simulink library "inSOMANET"  (R2016b)
settings: Solver=VariableStepAuto  StartTime=0.0  StopTime=10.0  RelTol=1e-3
libraries: ConversionsLibrary x28, xpcethercatlib x12
settings Model: Creator=Nathan  LastModifiedBy=MARCH

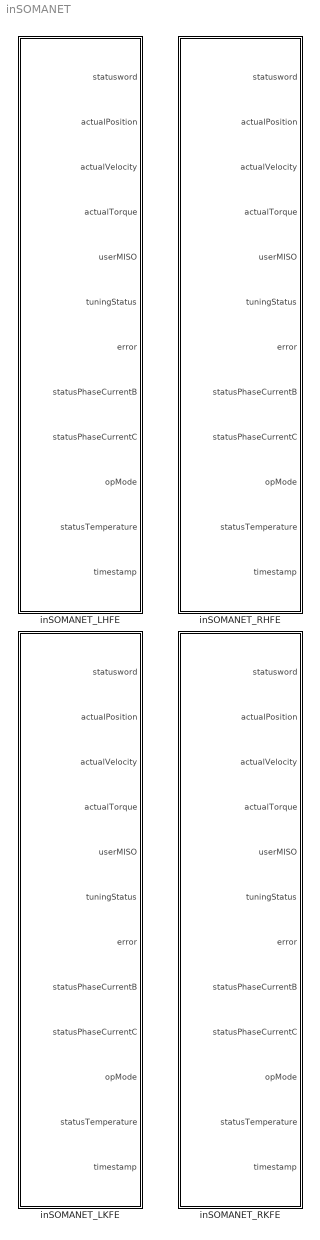
== system inSOMANET ==
  inSOMANET_LHFE : Subsystem
  inSOMANET_LKFE : Subsystem
  inSOMANET_RHFE : Subsystem
  inSOMANET_RKFE : Subsystem

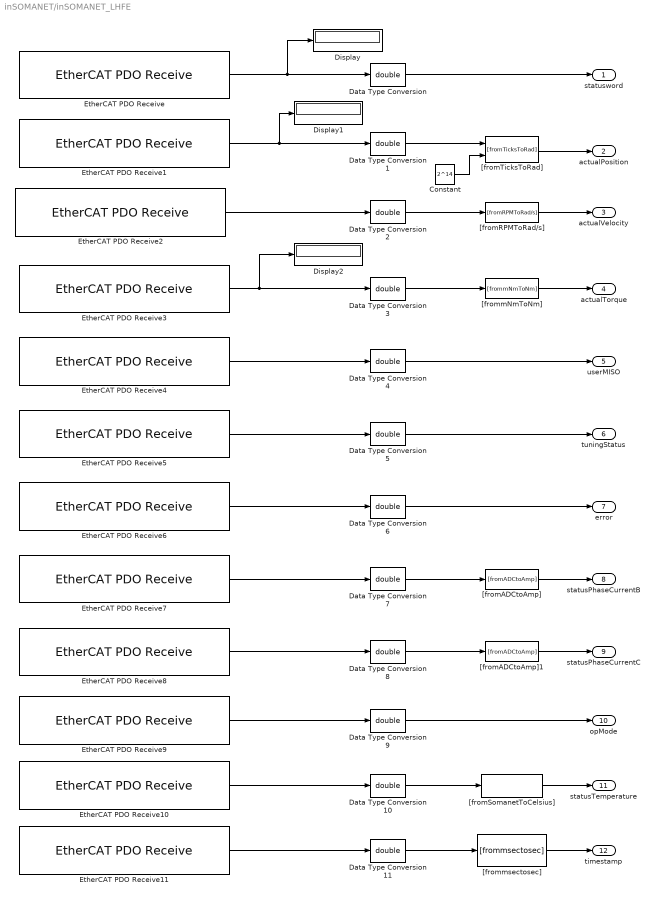
== system inSOMANET/inSOMANET_LHFE ==
  Constant : Constant  Value=2^14
  Data Type Conversion{,1..11} (12 alike) : DataTypeConversion  OutDataTypeStr=double
  Display : Display
  Display1 : Display
  Display2 : Display
  EtherCAT PDO Receive : xpcethercatlib/EtherCAT PDO Receive  Priority=2  sig_name=Drive 1 (CiA402 Motor Control Device).Inputs.Statusword  sig_offset=208  sig_type=uint16  type_size=16  sig_dim=1  device_id=0  sample_time=0.002000
  EtherCAT PDO Receive1 : xpcethercatlib/EtherCAT PDO Receive  Priority=2  sig_name=Drive 1 (CiA402 Motor Control Device).Inputs.Position Value  sig_offset=232  sig_type=int32  type_size=32  sig_dim=1  device_id=0  sample_time=0.002000
  EtherCAT PDO Receive10 : xpcethercatlib/EtherCAT PDO Receive  Priority=2  sig_name=Drive 1 (CiA402 Motor Control Device).Inputs.Core temperature  sig_offset=616  sig_type=int16  type_size=16  sig_dim=1  device_id=0  sample_time=0.002000
  EtherCAT PDO Receive11 : xpcethercatlib/EtherCAT PDO Receive  Priority=2  sig_name=Drive 1 (CiA402 Motor Control Device).Inputs.Timestamp  sig_offset=536  sig_type=uint32  type_size=32  sig_dim=1  device_id=0  sample_time=0.002000
  EtherCAT PDO Receive2 : xpcethercatlib/EtherCAT PDO Receive  Priority=2  sig_name=Drive 1 (CiA402 Motor Control Device).Inputs.Velocity Value  sig_offset=264  sig_type=int32  type_size=32  sig_dim=1  device_id=0  sample_time=0.002000
  EtherCAT PDO Receive3 : xpcethercatlib/EtherCAT PDO Receive  Priority=2  sig_name=Drive 1 (CiA402 Motor Control Device).Inputs.Torque Value  sig_offset=296  sig_type=int16  type_size=16  sig_dim=1  device_id=0  sample_time=0.002000
  EtherCAT PDO Receive4 : xpcethercatlib/EtherCAT PDO Receive  Priority=2  sig_name=Drive 1 (CiA402 Motor Control Device).Inputs.User MISO  sig_offset=504  sig_type=uint32  type_size=32  sig_dim=1  device_id=0  sample_time=0.002000
  EtherCAT PDO Receive5 : xpcethercatlib/EtherCAT PDO Receive  Priority=2  sig_name=Drive 1 (CiA402 Motor Control Device).Inputs.Tuning status  sig_offset=440  sig_type=uint32  type_size=32  sig_dim=1  device_id=0  sample_time=0.002000
  EtherCAT PDO Receive6 : xpcethercatlib/EtherCAT PDO Receive  Priority=2  sig_name=Drive 1 (CiA402 Motor Control Device).Inputs.Error code  sig_offset=568  sig_type=uint16  type_size=16  sig_dim=1  device_id=0  sample_time=0.002000
  EtherCAT PDO Receive7 : xpcethercatlib/EtherCAT PDO Receive  Priority=2  sig_name=Drive 1 (CiA402 Motor Control Device).Inputs.Instantaneous Phase B current  sig_offset=584  sig_type=int16  type_size=16  sig_dim=1  device_id=0  sample_time=0.002000
  EtherCAT PDO Receive8 : xpcethercatlib/EtherCAT PDO Receive  Priority=2  sig_name=Drive 1 (CiA402 Motor Control Device).Inputs.Instantaneous Phase C current  sig_offset=600  sig_type=int16  type_size=16  sig_dim=1  device_id=0  sample_time=0.002000
  EtherCAT PDO Receive9 : xpcethercatlib/EtherCAT PDO Receive  Priority=2  sig_name=Drive 1 (CiA402 Motor Control Device).Inputs.Op Mode Display  sig_offset=224  sig_type=int8  type_size=8  sig_dim=1  device_id=0  sample_time=0.002000
  "[fromADCtoAmp]" : ConversionsLibrary/[fromADCtoAmp]
  "[fromADCtoAmp]1" : ConversionsLibrary/[fromADCtoAmp]
  "[fromRPMToRad/s]" : ConversionsLibrary/[fromRPMToRad//s]
  "[fromSomanetToCelsius]" : ConversionsLibrary/[fromSomanetToCelsius]
  "[fromTicksToRad]" : ConversionsLibrary/[fromTicksToRad]
  "[frommNmToNm]" : ConversionsLibrary/[frommNmToNm]
  "[frommsectosec]" : ConversionsLibrary/[frommsectosec]
  statusword : Outport
  actualPosition : Outport  Port=2
  actualVelocity : Outport  Port=3
  actualTorque : Outport  Port=4
  userMISO : Outport  Port=5
  tuningStatus : Outport  Port=6
  error : Outport  Port=7
  statusPhaseCurrentB : Outport  Port=8
  statusPhaseCurrentC : Outport  Port=9
  opMode : Outport  Port=10
  statusTemperature : Outport  Port=11
  timestamp : Outport  Port=12
  wires:
  EtherCAT PDO Receive11/1 -> Data Type Conversion11/1
  EtherCAT PDO Receive10/1 -> Data Type Conversion10/1
  EtherCAT PDO Receive9/1 -> Data Type Conversion9/1
  EtherCAT PDO Receive8/1 -> Data Type Conversion8/1
  EtherCAT PDO Receive7/1 -> Data Type Conversion7/1
  EtherCAT PDO Receive6/1 -> Data Type Conversion6/1
  EtherCAT PDO Receive5/1 -> Data Type Conversion5/1
  EtherCAT PDO Receive4/1 -> Data Type Conversion4/1
  EtherCAT PDO Receive3/1 -> Data Type Conversion3/1, Display2/1
  EtherCAT PDO Receive2/1 -> Data Type Conversion2/1
  EtherCAT PDO Receive1/1 -> Data Type Conversion1/1, Display1/1
  EtherCAT PDO Receive/1 -> Data Type Conversion/1, Display/1
  Data Type Conversion/1 -> statusword/1
  Data Type Conversion11/1 -> "[frommsectosec]"/1
  Data Type Conversion10/1 -> "[fromSomanetToCelsius]"/1
  Data Type Conversion9/1 -> opMode/1
  Data Type Conversion8/1 -> "[fromADCtoAmp]1"/1
  Data Type Conversion7/1 -> "[fromADCtoAmp]"/1
  Data Type Conversion6/1 -> error/1
  Data Type Conversion5/1 -> tuningStatus/1
  Data Type Conversion4/1 -> userMISO/1
  Data Type Conversion3/1 -> "[frommNmToNm]"/1
  Data Type Conversion2/1 -> "[fromRPMToRad/s]"/1
  "[frommsectosec]"/1 -> timestamp/1
  "[fromSomanetToCelsius]"/1 -> statusTemperature/1
  "[fromADCtoAmp]1"/1 -> statusPhaseCurrentC/1
  "[fromADCtoAmp]"/1 -> statusPhaseCurrentB/1
  "[frommNmToNm]"/1 -> actualTorque/1
  "[fromRPMToRad/s]"/1 -> actualVelocity/1
  "[fromTicksToRad]"/1 -> actualPosition/1
  Data Type Conversion1/1 -> "[fromTicksToRad]"/1
  Constant/1 -> "[fromTicksToRad]"/2

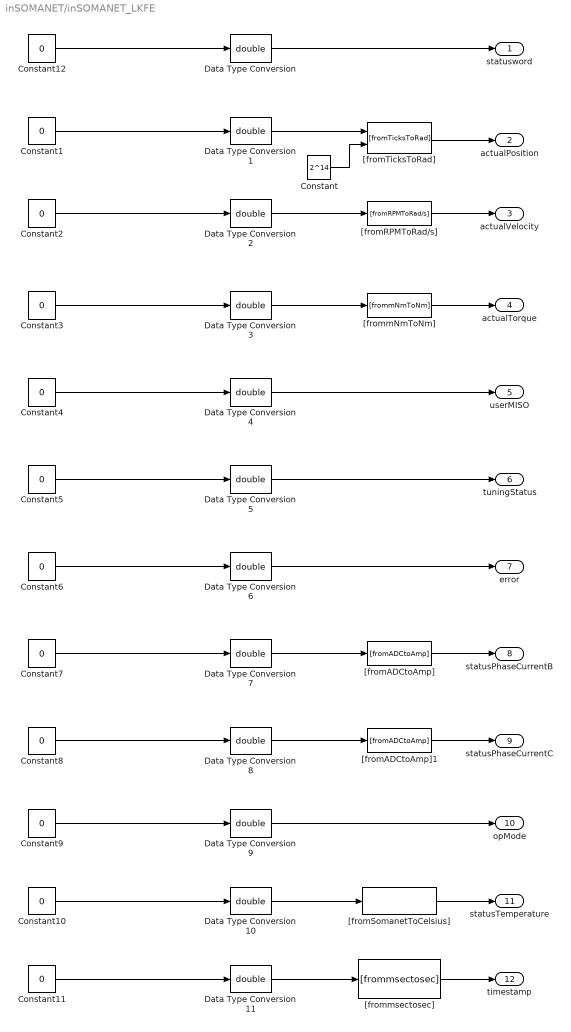
== system inSOMANET/inSOMANET_LKFE ==
  Constant : Constant  Value=2^14
  Constant{1..12} (12 alike) : Constant  Value=0
  Data Type Conversion{,1..11} (12 alike) : DataTypeConversion  OutDataTypeStr=double
  "[fromADCtoAmp]" : ConversionsLibrary/[fromADCtoAmp]
  "[fromADCtoAmp]1" : ConversionsLibrary/[fromADCtoAmp]
  "[fromRPMToRad/s]" : ConversionsLibrary/[fromRPMToRad//s]
  "[fromSomanetToCelsius]" : ConversionsLibrary/[fromSomanetToCelsius]
  "[fromTicksToRad]" : ConversionsLibrary/[fromTicksToRad]
  "[frommNmToNm]" : ConversionsLibrary/[frommNmToNm]
  "[frommsectosec]" : ConversionsLibrary/[frommsectosec]
  statusword : Outport
  actualPosition : Outport  Port=2
  actualVelocity : Outport  Port=3
  actualTorque : Outport  Port=4
  userMISO : Outport  Port=5
  tuningStatus : Outport  Port=6
  error : Outport  Port=7
  statusPhaseCurrentB : Outport  Port=8
  statusPhaseCurrentC : Outport  Port=9
  opMode : Outport  Port=10
  statusTemperature : Outport  Port=11
  timestamp : Outport  Port=12
  wires:
  Constant11/1 -> Data Type Conversion11/1
  Constant10/1 -> Data Type Conversion10/1
  Constant9/1 -> Data Type Conversion9/1
  Constant8/1 -> Data Type Conversion8/1
  Constant7/1 -> Data Type Conversion7/1
  Constant6/1 -> Data Type Conversion6/1
  Constant5/1 -> Data Type Conversion5/1
  Constant4/1 -> Data Type Conversion4/1
  Constant3/1 -> Data Type Conversion3/1
  Constant2/1 -> Data Type Conversion2/1
  Constant1/1 -> Data Type Conversion1/1
  Constant12/1 -> Data Type Conversion/1
  Data Type Conversion/1 -> statusword/1
  Data Type Conversion11/1 -> "[frommsectosec]"/1
  Data Type Conversion10/1 -> "[fromSomanetToCelsius]"/1
  Data Type Conversion9/1 -> opMode/1
  Data Type Conversion8/1 -> "[fromADCtoAmp]1"/1
  Data Type Conversion7/1 -> "[fromADCtoAmp]"/1
  Data Type Conversion6/1 -> error/1
  Data Type Conversion5/1 -> tuningStatus/1
  Data Type Conversion4/1 -> userMISO/1
  Data Type Conversion3/1 -> "[frommNmToNm]"/1
  Data Type Conversion2/1 -> "[fromRPMToRad/s]"/1
  "[frommsectosec]"/1 -> timestamp/1
  "[fromSomanetToCelsius]"/1 -> statusTemperature/1
  "[fromADCtoAmp]1"/1 -> statusPhaseCurrentC/1
  "[fromADCtoAmp]"/1 -> statusPhaseCurrentB/1
  "[frommNmToNm]"/1 -> actualTorque/1
  "[fromRPMToRad/s]"/1 -> actualVelocity/1
  "[fromTicksToRad]"/1 -> actualPosition/1
  Data Type Conversion1/1 -> "[fromTicksToRad]"/1
  Constant/1 -> "[fromTicksToRad]"/2

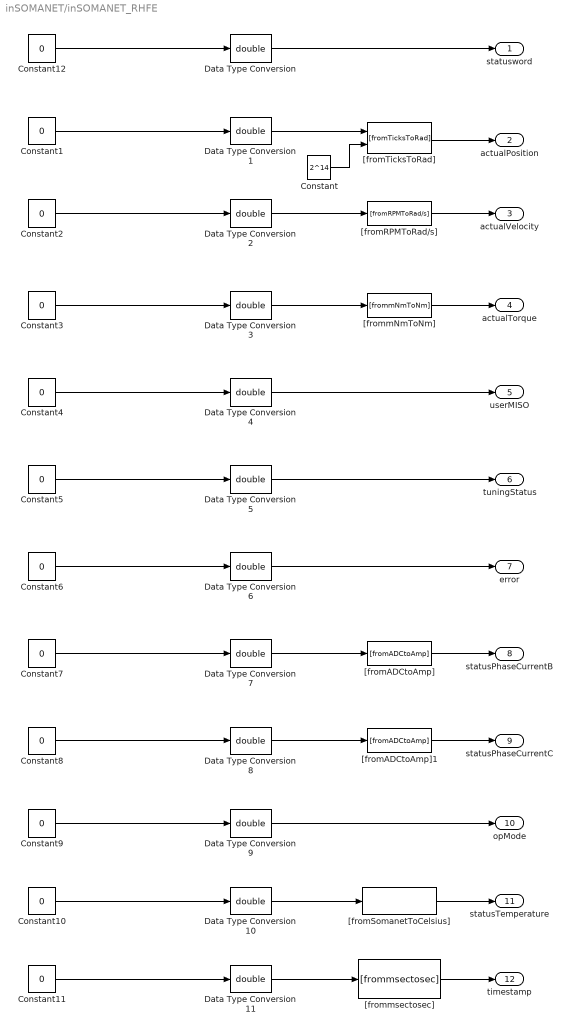
== system inSOMANET/inSOMANET_RHFE ==
  Constant : Constant  Value=2^14
  Constant{1..12} (12 alike) : Constant  Value=0
  Data Type Conversion{,1..11} (12 alike) : DataTypeConversion  OutDataTypeStr=double
  "[fromADCtoAmp]" : ConversionsLibrary/[fromADCtoAmp]
  "[fromADCtoAmp]1" : ConversionsLibrary/[fromADCtoAmp]
  "[fromRPMToRad/s]" : ConversionsLibrary/[fromRPMToRad//s]
  "[fromSomanetToCelsius]" : ConversionsLibrary/[fromSomanetToCelsius]
  "[fromTicksToRad]" : ConversionsLibrary/[fromTicksToRad]
  "[frommNmToNm]" : ConversionsLibrary/[frommNmToNm]
  "[frommsectosec]" : ConversionsLibrary/[frommsectosec]
  statusword : Outport
  actualPosition : Outport  Port=2
  actualVelocity : Outport  Port=3
  actualTorque : Outport  Port=4
  userMISO : Outport  Port=5
  tuningStatus : Outport  Port=6
  error : Outport  Port=7
  statusPhaseCurrentB : Outport  Port=8
  statusPhaseCurrentC : Outport  Port=9
  opMode : Outport  Port=10
  statusTemperature : Outport  Port=11
  timestamp : Outport  Port=12
  wires:
  Constant11/1 -> Data Type Conversion11/1
  Constant10/1 -> Data Type Conversion10/1
  Constant9/1 -> Data Type Conversion9/1
  Constant8/1 -> Data Type Conversion8/1
  Constant7/1 -> Data Type Conversion7/1
  Constant6/1 -> Data Type Conversion6/1
  Constant5/1 -> Data Type Conversion5/1
  Constant4/1 -> Data Type Conversion4/1
  Constant3/1 -> Data Type Conversion3/1
  Constant2/1 -> Data Type Conversion2/1
  Constant1/1 -> Data Type Conversion1/1
  Constant12/1 -> Data Type Conversion/1
  Data Type Conversion/1 -> statusword/1
  Data Type Conversion11/1 -> "[frommsectosec]"/1
  Data Type Conversion10/1 -> "[fromSomanetToCelsius]"/1
  Data Type Conversion9/1 -> opMode/1
  Data Type Conversion8/1 -> "[fromADCtoAmp]1"/1
  Data Type Conversion7/1 -> "[fromADCtoAmp]"/1
  Data Type Conversion6/1 -> error/1
  Data Type Conversion5/1 -> tuningStatus/1
  Data Type Conversion4/1 -> userMISO/1
  Data Type Conversion3/1 -> "[frommNmToNm]"/1
  Data Type Conversion2/1 -> "[fromRPMToRad/s]"/1
  "[frommsectosec]"/1 -> timestamp/1
  "[fromSomanetToCelsius]"/1 -> statusTemperature/1
  "[fromADCtoAmp]1"/1 -> statusPhaseCurrentC/1
  "[fromADCtoAmp]"/1 -> statusPhaseCurrentB/1
  "[frommNmToNm]"/1 -> actualTorque/1
  "[fromRPMToRad/s]"/1 -> actualVelocity/1
  "[fromTicksToRad]"/1 -> actualPosition/1
  Data Type Conversion1/1 -> "[fromTicksToRad]"/1
  Constant/1 -> "[fromTicksToRad]"/2

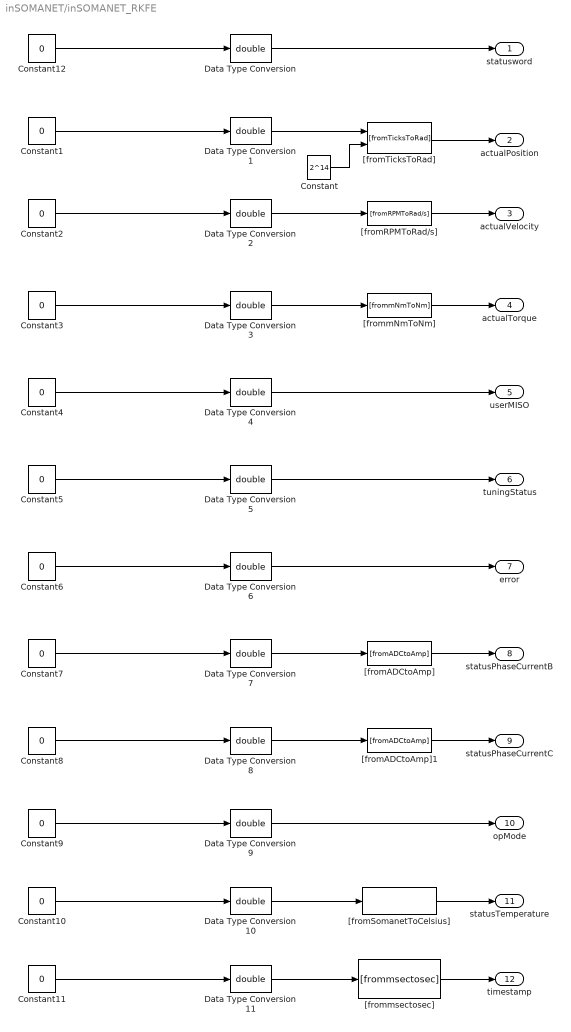
== system inSOMANET/inSOMANET_RKFE ==
  Constant : Constant  Value=2^14
  Constant{1..12} (12 alike) : Constant  Value=0
  Data Type Conversion{,1..11} (12 alike) : DataTypeConversion  OutDataTypeStr=double
  "[fromADCtoAmp]" : ConversionsLibrary/[fromADCtoAmp]
  "[fromADCtoAmp]1" : ConversionsLibrary/[fromADCtoAmp]
  "[fromRPMToRad/s]" : ConversionsLibrary/[fromRPMToRad//s]
  "[fromSomanetToCelsius]" : ConversionsLibrary/[fromSomanetToCelsius]
  "[fromTicksToRad]" : ConversionsLibrary/[fromTicksToRad]
  "[frommNmToNm]" : ConversionsLibrary/[frommNmToNm]
  "[frommsectosec]" : ConversionsLibrary/[frommsectosec]
  statusword : Outport
  actualPosition : Outport  Port=2
  actualVelocity : Outport  Port=3
  actualTorque : Outport  Port=4
  userMISO : Outport  Port=5
  tuningStatus : Outport  Port=6
  error : Outport  Port=7
  statusPhaseCurrentB : Outport  Port=8
  statusPhaseCurrentC : Outport  Port=9
  opMode : Outport  Port=10
  statusTemperature : Outport  Port=11
  timestamp : Outport  Port=12
  wires:
  Constant11/1 -> Data Type Conversion11/1
  Constant10/1 -> Data Type Conversion10/1
  Constant9/1 -> Data Type Conversion9/1
  Constant8/1 -> Data Type Conversion8/1
  Constant7/1 -> Data Type Conversion7/1
  Constant6/1 -> Data Type Conversion6/1
  Constant5/1 -> Data Type Conversion5/1
  Constant4/1 -> Data Type Conversion4/1
  Constant3/1 -> Data Type Conversion3/1
  Constant2/1 -> Data Type Conversion2/1
  Constant1/1 -> Data Type Conversion1/1
  Constant12/1 -> Data Type Conversion/1
  Data Type Conversion/1 -> statusword/1
  Data Type Conversion11/1 -> "[frommsectosec]"/1
  Data Type Conversion10/1 -> "[fromSomanetToCelsius]"/1
  Data Type Conversion9/1 -> opMode/1
  Data Type Conversion8/1 -> "[fromADCtoAmp]1"/1
  Data Type Conversion7/1 -> "[fromADCtoAmp]"/1
  Data Type Conversion6/1 -> error/1
  Data Type Conversion5/1 -> tuningStatus/1
  Data Type Conversion4/1 -> userMISO/1
  Data Type Conversion3/1 -> "[frommNmToNm]"/1
  Data Type Conversion2/1 -> "[fromRPMToRad/s]"/1
  "[frommsectosec]"/1 -> timestamp/1
  "[fromSomanetToCelsius]"/1 -> statusTemperature/1
  "[fromADCtoAmp]1"/1 -> statusPhaseCurrentC/1
  "[fromADCtoAmp]"/1 -> statusPhaseCurrentB/1
  "[frommNmToNm]"/1 -> actualTorque/1
  "[fromRPMToRad/s]"/1 -> actualVelocity/1
  "[fromTicksToRad]"/1 -> actualPosition/1
  Data Type Conversion1/1 -> "[fromTicksToRad]"/1
  Constant/1 -> "[fromTicksToRad]"/2
